simulink model "unifier_obm_wrapper"  (R2023b)
settings: Solver=ode1  StartTime=0.0  StopTime=1/500  FixedStep=1/500  RelTol=1e-3
libraries: unifier_obm x1
settings Model: Creator=johannes  LastModifiedBy=johannes

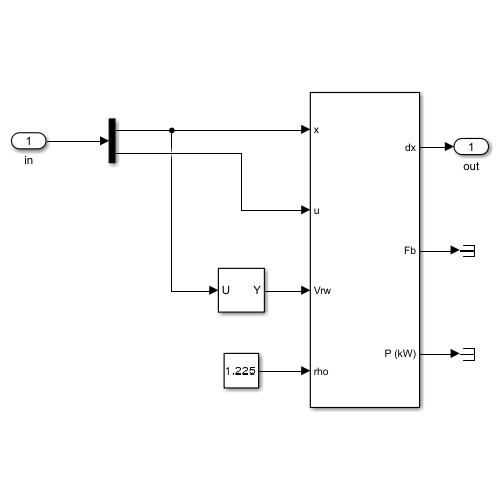
[thumbnail: Simulink's stored preview of the top-level diagram]
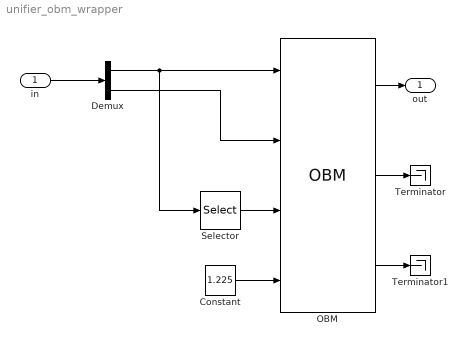
== system unifier_obm_wrapper ==
  in : Inport
  Constant : Constant  Value=1.225
  Demux : Demux  Outputs=[12,20]
  OBM : unifier_obm/OBM  SystemSampleTime=-1  VariantActivationTime=update diagram  AllowFlexibleInterface=on  Latency=0  AutoFrameSizeCalculation=off
  Selector : Selector  InputPortWidth=12  IndexOptions=Index vector (dialog)  Indices=[4,5,6]  OutputSizes=1
  Terminator : Terminator
  Terminator1 : Terminator
  out : Outport
  wires:
  Demux/1 -> Selector/1, OBM/1
  Demux/2 -> OBM/2
  Selector/1 -> OBM/3
  Constant/1 -> OBM/4
  OBM/2 -> Terminator/1
  OBM/3 -> Terminator1/1
  OBM/1 -> out/1
  in/1 -> Demux/1
